simulink model "maglev_quick_start"  (Simulink 9.2)
settings: Solver=ode1  StartTime=0.0  StopTime=inf  FixedStep=0.002  RelTol=1e-3  EnableMultiTasking=on
PostLoadFcn:
  | qc_set_target_type(getConfigSet(bdroot, 'QUARC Default Target Configuration'));
undefined symbols (not defined in the file or in its folder): HIL
libraries: quarc_library x3
settings Model: Creator=MLevis  LastModifiedBy=p1805627  SimulationMode=external  ExtModeTrigDuration=5000
settings SolverCC: PositivePriorityOrder=on
settings OptimizationCC: ExpressionDepthLimit=2147483647  InitFltsAndDblsToZero=on
settings DebuggingCC: SaveWithParameterizedLinksMsg=none  SolverPrmCheckMsg=warning  MultiTaskDSMMsg=warning  MultiTaskCondExecSysMsg=none
settings RTWCC: SystemTargetFile=quarc_win64.tlc  TemplateMakefile=quarc_default_tmf  Description=QUARC Win64 Target
settings STFCustomTargetCC: TargetPreCompLibLocation=C:\PROGRA~3\QUARC\lib\2011a\win64\release  ConcurrentExecutionCompliant=on  GeneratePreprocessorConditionals=Disable all  CPPClassGenCompliant=on  SystemTargetFile=quarc_win64.tlc
settings GRTTargetCC: TargetPreCompLibLocation=C:\PROGRA~3\QUARC\lib\2018b\win64\release  ParMdlRefBuildCompliant=off  CompOptLevelCompliant=off  MatFileLogging=off  UseToolchainInfoCompliant=off  ExtMode=on  ExtModeMexFile=quarc_comm

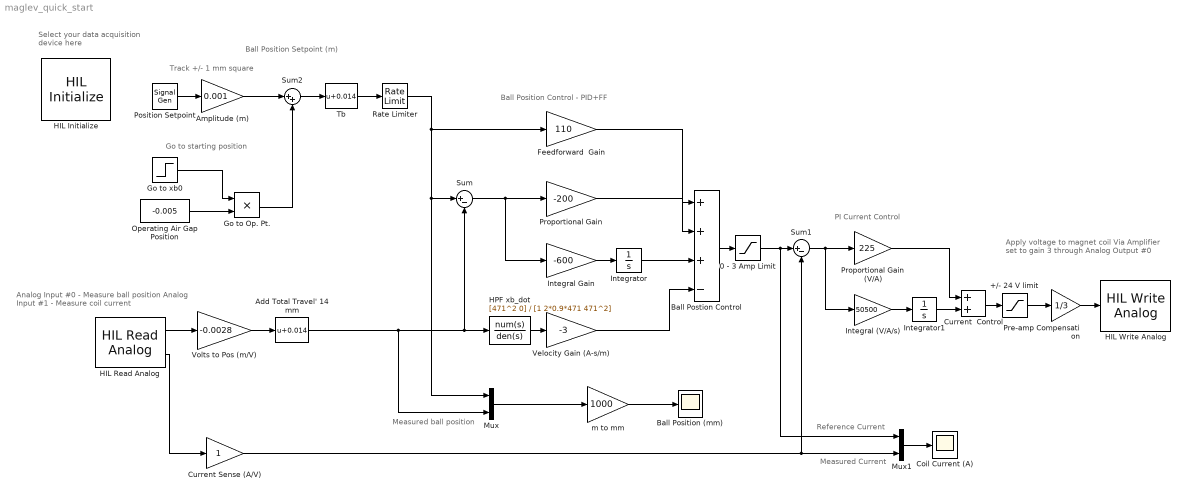
== system maglev_quick_start ==
  note: Select  your data
      | acquisition device here
  note: Apply voltage to magnet coil
      | Via Amplifier set to gain 3 through
      | Analog Output #0
  note: Analog Input #0 - Measure ball position
      | Analog Input #1 - Measure coil current
  note: Ball Position Control - PID+FF
  note: PI Current Control
  note: Ball Position Setpoint (m)
  note: Track +/- 1 mm square
  note: Go to starting position
  note: Reference Current
  note: Measured Current
  note: Measured ball position
  " +/- 24 V limit" : Saturate  UpperLimit=24  LowerLimit=-24
  0 - 3 Amp Limit : Saturate  UpperLimit=3  LowerLimit=0
  Add Total Travel' 14 mm : Bias  Bias=0.014
  Amplitude (m) : Gain  Gain=0.001  SaturateOnIntegerOverflow=on  OutDataTypeStr=Inherit: Same as input  ParamDataTypeStr=Inherit: Same as input
  Ball Postion Control : Sum  Inputs=+++-
  Ball Position (mm) : Scope
  "Coil Current (A) " : Scope
  Current  Control : Sum
  "Current Sense (A/V) " : Gain
  Feedforward  Gain : Gain  Gain=110
  Go to Op. Pt. : Product  RndMeth=Zero
  Go to xb0 : Step  Time=2  SampleTime=0
  HIL Initialize : quarc_library/Data Acquisition/Generic/Configuration/HIL Initialize  object_name=HIL-1  board_type=q2_usb  board_number=0  board_options=d0=digital;d1=digital;led=auto;update_rate=normal;decimation=1  exclusive=off  active=off  hardware_clocks=[0]  clock_modes=[]  initial_clock_frequencies=[]  set_clock_params_at_start=off  set_clock_params_at_switch_in=off  set_clock_frequencies_at_start=off  set_clock_frequencies_at_switch_in=off  analog_input_channels=[0:1]  analog_input_configurations=[]  analog_input_maximums=10  analog_input_minimums=-10  set_analog_input_params_at_start=on  set_analog_input_params_at_switch_in=off  analog_output_channels=[0:1]  analog_output_maximums=10  analog_output_minimums=-10  initial_analog_outputs=[0]  final_analog_outputs=[0]  watchdog_analog_outputs=0  set_analog_output_params_at_start=on  set_analog_output_params_at_switch_in=off  set_analog_outputs_at_start=on  set_analog_outputs_at_switch_in=off  set_analog_outputs_at_terminate=on  set_analog_outputs_at_switch_out=off  set_analog_outputs_on_watchdog=off  digital_input_channels=[]  digital_output_channels=[]  digital_output_configuration=[]  initial_digital_outputs=[1]  final_digital_outputs=[1]  watchdog_digital_outputs=[1]  set_digital_output_params_at_start=off  set_digital_output_params_at_switch_in=off  set_digital_outputs_at_start=on  set_digital_outputs_at_switch_in=off  set_digital_outputs_at_terminate=on  set_digital_outputs_at_switch_out=off  set_digital_outputs_on_watchdog=off  encoder_channels=[0:1]  quadrature=[4]  encoder_filter_frequency=[]  initial_encoder_counts=[0]  set_encoder_params_at_start=on  set_encoder_params_at_switch_in=off  set_encoder_counts_at_start=on  set_encoder_counts_at_switch_in=off  pwm_channels=[]  pwm_modes=[0]  pwm_frequency=1/0.020  pwm_configuration=[]  pwm_alignment=[]  pwm_polarity=[]  pwm_leading_deadband=[]  pwm_trailing_deadband=[]  initial_pwm_outputs=[0]  final_pwm_outputs=[0]  watchdog_pwm_outputs=[0]  set_pwm_params_at_start=on  set_pwm_params_at_switch_in=off  set_pwm_outputs_at_start=on  set_pwm_outputs_at_switch_in=off  set_pwm_outputs_at_terminate=on  set_pwm_outputs_at_switch_out=off  set_pwm_outputs_on_watchdog=off  other_output_channels=[]  initial_other_outputs=[]  final_other_outputs=[]  watchdog_other_outputs=[]  set_other_outputs_at_start=off  set_other_outputs_at_switch_in=off  set_other_outputs_at_terminate=off  set_other_outputs_at_switch_out=off  set_other_outputs_on_watchdog=off
  HIL Read Analog : quarc_library/Data Acquisition/Generic/Immediate I//O/HIL Read Analog  object_name=HIL-1  channels=[0:1]  sample_time=qc_get_step_size  active=on  vector_output=off
  HIL Write Analog : quarc_library/Data Acquisition/Generic/Immediate I//O/HIL Write Analog  object_name=HIL-1  channels=0  sample_time=-1  active=off  vector_input=off
  HPF xb_dot : TransferFcn  Numerator=[471^2 0]  Denominator=[1 2*0.9*471 471^2]
  "Integral (V/A/s) " : Gain  Gain=50500
  "Integral Gain " : Gain  Gain=-600
  Integrator : Integrator  LimitOutput=on  UpperSaturationLimit=3  LowerSaturationLimit=-3
  Integrator1 : Integrator  LimitOutput=on  UpperSaturationLimit=3  LowerSaturationLimit=-3
  Mux : Mux  Inputs=2
  Mux1 : Mux  Inputs=2
  Operating Air Gap Position : Constant  Value=-0.005
  Position Setpoint : SignalGenerator  WaveForm=square  Frequency=.25
  Pre-amp Compensation : Gain  Gain=1/3
  Proportional Gain : Gain  Gain=-200
  "Proportional Gain (V/A) " : Gain  Gain=225
  Rate Limiter : RateLimiter  RisingSlewLimit=5e-3  FallingSlewLimit=-5e-3  SampleTimeMode=inherited
  Sum : Sum  Inputs=|+-
  Sum1 : Sum  Inputs=|+-
  Sum2 : Sum  Inputs=|++
  Tb : Bias  Bias=0.014
  "Velocity Gain (A-s/m) " : Gain  Gain=-3
  "Volts to Pos (m/V) " : Gain  Gain=-0.0028
  "m to mm " : Gain  Gain=1000
  wires:
  0 - 3 Amp Limit/1 -> Sum1/1, Mux1/1
  HIL Read Analog/1 -> "Volts to Pos (m/V) "/1
  Ball Postion Control/1 -> 0 - 3 Amp Limit/1
  Feedforward  Gain/1 -> Ball Postion Control/1
  "Integral Gain "/1 -> Integrator/1
  Proportional Gain/1 -> Ball Postion Control/2
  Integrator/1 -> Ball Postion Control/3
  Sum/1 -> Proportional Gain/1, "Integral Gain "/1
  Add Total Travel' 14 mm/1 -> Mux/2, Sum/2, HPF xb_dot/1
  Mux/1 -> "m to mm "/1
  "Current Sense (A/V) "/1 -> Sum1/2, Mux1/2
  HPF xb_dot/1 -> "Velocity Gain (A-s/m) "/1
  "Velocity Gain (A-s/m) "/1 -> Ball Postion Control/4
  Sum1/1 -> "Proportional Gain (V/A) "/1, "Integral (V/A/s) "/1
  "Integral (V/A/s) "/1 -> Integrator1/1
  Integrator1/1 -> Current  Control/2
  "Proportional Gain (V/A) "/1 -> Current  Control/1
  Current  Control/1 -> " +/- 24 V limit"/1
  " +/- 24 V limit"/1 -> Pre-amp Compensation/1
  Pre-amp Compensation/1 -> HIL Write Analog/1
  Mux1/1 -> "Coil Current (A) "/1
  Rate Limiter/1 -> Feedforward  Gain/1, Mux/1, Sum/1
  Position Setpoint/1 -> Amplitude (m)/1
  Sum2/1 -> Tb/1
  Operating Air Gap Position/1 -> Go to Op. Pt./2
  Go to xb0/1 -> Go to Op. Pt./1
  Tb/1 -> Rate Limiter/1
  "m to mm "/1 -> Ball Position (mm)/1
  HIL Read Analog/2 -> "Current Sense (A/V) "/1
  Go to Op. Pt./1 -> Sum2/2
  Amplitude (m)/1 -> Sum2/1
  "Volts to Pos (m/V) "/1 -> Add Total Travel' 14 mm/1
